simulink model "model"  (R2020a)
settings: Solver=FixedStepAuto  StartTime=0.0  StopTime=200  FixedStep=0.01  RelTol=1e-3
values from neighbouring files (symbols this model uses):
  A = zeros(5,5)    [init_test.m]
  b = 2*10^5    (= 200000)    [init_test.m]
  d1 = 2    [init_test.m]
  d2 = 3    [init_test.m]
  d3 = 3    [init_test.m]
  d4 = 2    [init_test.m]
  fleet_vel = 20    [init_test.m]
  h10 = -0.8    [init_test.m]
  h20 = h10*2    (= -1.6)    [init_test.m]
  h30 = h10*3    (= -2.4)    [init_test.m]
  h40 = h10*4    (= -3.2)    [init_test.m]
  k1 = 1.7*10^5    (= 170000)    [init_test.m]
  k2 = 1.8*10^5    (= 180000)    [init_test.m]
  k3 = 1.8*10^5    (= 180000)    [init_test.m]
  k4 = 1.2*10^5    (= 120000)    [init_test.m]
  M = 1200    [init_test.m]
  n0_init = [0 20]    [init_test.m]
  n1_init = [-10 0]    [init_test.m]
  n2_init = [-20 0]    [init_test.m]
  n3_init = [-30 0]    [init_test.m]
  n4_init = [-40 0]    [init_test.m]
  noise = 1    [init_test.m]
  u0 = 0    [init_test.m]
settings Model: Creator=mic-ciciolla  LastModifiedBy=mic-ciciolla

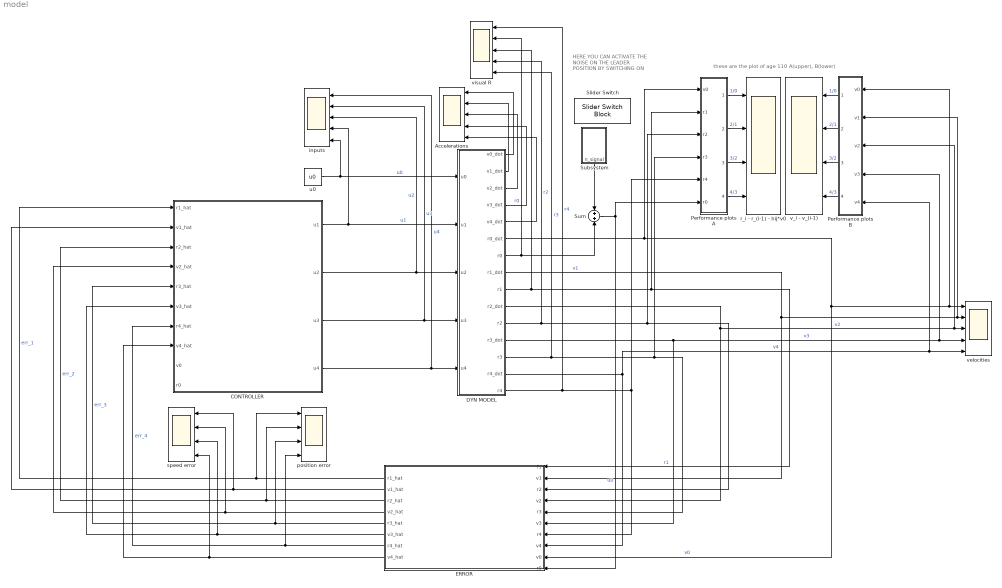
== system model ==
  note: these are the plot of age 110 A(upper), B(lower)
  note: HERE YOU CAN ACTIVATE THE NOISE ON THE LEADER POSITION BY SWITCHING ON
  Accelerations : Scope  NumInputPorts=5
  CONTROLLER : Subsystem
  DYN MODEL : Subsystem
  ERROR : Subsystem
  Performance plots A : Subsystem
  Performance plots B : Subsystem
  Slider Switch : SliderSwitchBlock
      settings: Values={{'Off', 'On'}, [0 1]}
  Subsystem : Subsystem
      settings: PortSchema="{\"entries\":[{\"content\":{\"sides\":[{\"content\":{\"connectorIds\":[]},\"type\":\"ConnectorPlacement.EquallySpacedRectSide\",\"uuid\":\"16fede81-657e-45c1-a9ae-d81e864610a5\"},{\"content\":{\"connectorIds\":[],\"side\":\"RIGHT\"},\"type\":\"ConnectorPlacement.EquallySpacedRectSide\",\"uuid\":\"97676902-59d3-4a36-b26f-8c9a1bb8a23e\"},{\"content\":{\"connectorIds\":[],\"side\":\"TOP\"},\"type\":\"ConnectorPlacement.EquallySpacedRectSide\",\"uuid\":\"8e239925-b658-4eae-ba83-be624b434eda\"},{\"content\":{\"connectorIds\":[\"Out1\"],\"side\":\"BOTTOM\"},\"type\":\"ConnectorPlacement.EquallySpacedRectSide\",\"uuid\":\"030014d3-1c2a-45c6-8ce4-97b9acd07308\"}]},\"type\":\"ConnectorPlacement.EquallySpacedConnector\",\"uuid\":\"2f76814e-6954-4e9d-8491-731c603c8c68\"}],\"packageUris\":[\"http://schema.mathworks.com/mf0/Connector/19700101\"],\"version\":\"1.0\"}"
  Sum : Sum
  inputs : Scope  NumInputPorts=5
  position error : Scope  NumInputPorts=4
  r_i - r_(i-1) - hij*v0 : Scope  NumInputPorts=4
  speed error : Scope  NumInputPorts=4
  u0 : Constant  Value=u0
  v_i - v_(i-1) : Scope  NumInputPorts=4
  velocities : Scope  NumInputPorts=5
  visual R : Scope  NumInputPorts=5
  wires:
  DYN MODEL/9(r1) -> visual R/3, Performance plots A/2(r1), ERROR/1(r1)  "r1"
  DYN MODEL/8(r1_dot) -> Performance plots B/2(v1), velocities/2, ERROR/2(v1)  "v1"
  DYN MODEL/7(r0) -> Sum/2, visual R/2  "r0"
  DYN MODEL/6(r0_dot) -> Performance plots A/1(v0), ERROR/9(v0), Performance plots B/1(v0), velocities/1  "v0"
  DYN MODEL/11(r2) -> ERROR/3(r2), Performance plots A/3(r2), visual R/4  "r2"
  DYN MODEL/10(r2_dot) -> Performance plots B/3(v2), velocities/3, ERROR/4(v2)  "v2"
  DYN MODEL/13(r3) -> ERROR/5(r3), Performance plots A/4(r3), visual R/5  "r3"
  DYN MODEL/12(r3_dot) -> Performance plots B/4(v3), velocities/4, ERROR/6(v3)  "v3"
  DYN MODEL/15(r4) -> visual R/1, Performance plots A/5(r4), ERROR/7(r4)  "r4"
  DYN MODEL/14(r4_dot) -> velocities/5, Performance plots B/5(v4), ERROR/8(v4)  "v4"
  ERROR/1(r1_hat) -> position error/1, CONTROLLER/1(r1_hat)  "err_1"
  ERROR/2(v1_hat) -> CONTROLLER/2(v1_hat), speed error/1
  ERROR/3(r2_hat) -> position error/2, CONTROLLER/3(r2_hat)  "err_2"
  ERROR/4(v2_hat) -> CONTROLLER/4(v2_hat), speed error/2
  ERROR/5(r3_hat) -> position error/3, CONTROLLER/5(r3_hat)  "err_3"
  ERROR/6(v3_hat) -> speed error/3, CONTROLLER/6(v3_hat)
  ERROR/7(r4_hat) -> position error/4, CONTROLLER/7(r4_hat)  "err_4"
  ERROR/8(v4_hat) -> speed error/4, CONTROLLER/8(v4_hat)
  CONTROLLER/1(u1) -> inputs/4, DYN MODEL/2(u1)  "u1"
  CONTROLLER/2(u2) -> inputs/3, DYN MODEL/3(u2)  "u2"
  CONTROLLER/3(u3) -> inputs/2, DYN MODEL/4(u3)  "u3"
  CONTROLLER/4(u4) -> inputs/1, DYN MODEL/5(u4)  "u4"
  Performance plots B/1(veic 1/0) -> v_i - v_(i-1)/1  "1/0"
  Performance plots B/2(veic 2/1) -> v_i - v_(i-1)/2  "2/1"
  Performance plots B/4(veic 4/3) -> v_i - v_(i-1)/4  "4/3"
  Performance plots B/3(veic 3/2) -> v_i - v_(i-1)/3  "3/2"
  Performance plots A/4(veic 4/3) -> r_i - r_(i-1) - hij*v0/4  "4/3"
  Performance plots A/3(veic 3/2) -> r_i - r_(i-1) - hij*v0/3  "3/2"
  Performance plots A/1(veic 1/0) -> r_i - r_(i-1) - hij*v0/1  "1/0"
  Performance plots A/2(veic 2/1) -> r_i - r_(i-1) - hij*v0/2  "2/1"
  u0/1 -> inputs/5, DYN MODEL/1(u0)  "u0"
  Sum/1 -> ERROR/10(r0), Performance plots A/6(r0)  "u0"
  DYN MODEL/1(v0_dot) -> Accelerations/1
  DYN MODEL/2(v1_dot) -> Accelerations/2
  DYN MODEL/3(v2_dot) -> Accelerations/3
  DYN MODEL/4(v3_dot) -> Accelerations/4
  DYN MODEL/5(v4_dot) -> Accelerations/5
  Subsystem/1(n_signal) -> Sum/1

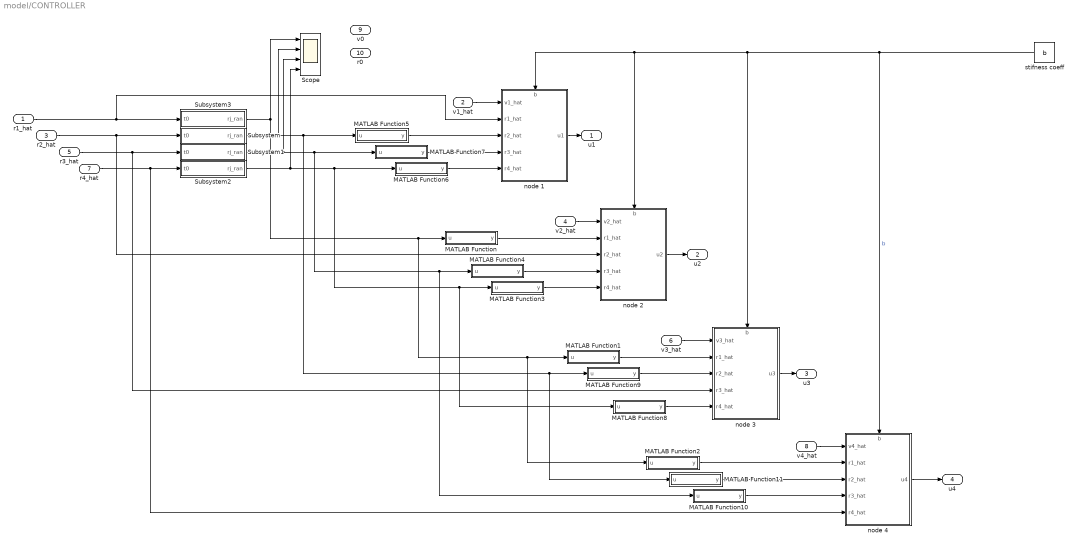
== system model/CONTROLLER ==
  r1_hat : Inport
  v1_hat : Inport  Port=2
  r2_hat : Inport  Port=3
  v2_hat : Inport  Port=4
  r3_hat : Inport  Port=5
  v3_hat : Inport  Port=6
  r4_hat : Inport  Port=7
  v4_hat : Inport  Port=8
  v0 : Inport  Port=9
  r0 : Inport  Port=10
  MATLAB Function : MATLAB Function  TreatAsAtomicUnit=on
  MATLAB Function1 : MATLAB Function  TreatAsAtomicUnit=on
  MATLAB Function10 : MATLAB Function  TreatAsAtomicUnit=on
  MATLAB Function11 : MATLAB Function  TreatAsAtomicUnit=on
  MATLAB Function2 : MATLAB Function  TreatAsAtomicUnit=on
  MATLAB Function3 : MATLAB Function  TreatAsAtomicUnit=on
  MATLAB Function4 : MATLAB Function  TreatAsAtomicUnit=on
  MATLAB Function5 : MATLAB Function  TreatAsAtomicUnit=on
  MATLAB Function6 : MATLAB Function  TreatAsAtomicUnit=on
  MATLAB Function7 : MATLAB Function  TreatAsAtomicUnit=on
  MATLAB Function8 : MATLAB Function  TreatAsAtomicUnit=on
  MATLAB Function9 : MATLAB Function  TreatAsAtomicUnit=on
  Scope : Scope  NumInputPorts=4
  Subsystem : Subsystem
  Subsystem1 : Subsystem
  Subsystem2 : Subsystem
  Subsystem3 : Subsystem
  node 1 : Subsystem
      settings: PortSchema="{\"entries\":[{\"content\":{\"sides\":[{\"content\":{\"connectorIds\":[\"In1\",\"In2\",\"In3\",\"In4\",\"In5\"]},\"type\":\"ConnectorPlacement.EquallySpacedRectSide\",\"uuid\":\"5e8ab726-83fb-4f3c-9500-0538f81a3a18\"},{\"content\":{\"connectorIds\":[\"Out1\"],\"side\":\"RIGHT\"},\"type\":\"ConnectorPlacement.EquallySpacedRectSide\",\"uuid\":\"1c3f6fdc-5897-44be-b75d-625b3a56e21f\"},{\"content\":{\"connectorIds\":[\"In6\"],\"side\":\"TOP\"},\"type\":\"ConnectorPlacement.EquallySpacedRectSide\",\"uuid\":\"dec3deb1-028d-4c92-801a-3054ae4cd420\"}]},\"type\":\"ConnectorPlacement.EquallySpacedConnector\",\"uuid\":\"f32b6f2a-1ac7-4706-92ec-1bae63a0d6a6\"}],\"packageUris\":[\"http://schema.mathworks.com/mf0/Connector/19700101\"],\"version\":\"1.0\"}"
  node 2 : Subsystem
      settings: PortSchema="{\"entries\":[{\"content\":{\"sides\":[{\"content\":{\"connectorIds\":[\"In1\",\"In2\",\"In3\",\"In4\",\"In5\"]},\"type\":\"ConnectorPlacement.EquallySpacedRectSide\",\"uuid\":\"5e8ab726-83fb-4f3c-9500-0538f81a3a18\"},{\"content\":{\"connectorIds\":[\"Out1\"],\"side\":\"RIGHT\"},\"type\":\"ConnectorPlacement.EquallySpacedRectSide\",\"uuid\":\"1c3f6fdc-5897-44be-b75d-625b3a56e21f\"},{\"content\":{\"connectorIds\":[\"In6\"],\"side\":\"TOP\"},\"type\":\"ConnectorPlacement.EquallySpacedRectSide\",\"uuid\":\"dec3deb1-028d-4c92-801a-3054ae4cd420\"}]},\"type\":\"ConnectorPlacement.EquallySpacedConnector\",\"uuid\":\"f32b6f2a-1ac7-4706-92ec-1bae63a0d6a6\"}],\"packageUris\":[\"http://schema.mathworks.com/mf0/Connector/19700101\"],\"version\":\"1.0\"}"
  node 3 : Subsystem
      settings: PortSchema="{\"entries\":[{\"content\":{\"sides\":[{\"content\":{\"connectorIds\":[\"In1\",\"In2\",\"In3\",\"In4\",\"In5\"]},\"type\":\"ConnectorPlacement.EquallySpacedRectSide\",\"uuid\":\"5e8ab726-83fb-4f3c-9500-0538f81a3a18\"},{\"content\":{\"connectorIds\":[\"Out1\"],\"side\":\"RIGHT\"},\"type\":\"ConnectorPlacement.EquallySpacedRectSide\",\"uuid\":\"1c3f6fdc-5897-44be-b75d-625b3a56e21f\"},{\"content\":{\"connectorIds\":[\"In6\"],\"side\":\"TOP\"},\"type\":\"ConnectorPlacement.EquallySpacedRectSide\",\"uuid\":\"dec3deb1-028d-4c92-801a-3054ae4cd420\"}]},\"type\":\"ConnectorPlacement.EquallySpacedConnector\",\"uuid\":\"f32b6f2a-1ac7-4706-92ec-1bae63a0d6a6\"}],\"packageUris\":[\"http://schema.mathworks.com/mf0/Connector/19700101\"],\"version\":\"1.0\"}"
  node 4 : Subsystem
      settings: PortSchema="{\"entries\":[{\"content\":{\"sides\":[{\"content\":{\"connectorIds\":[\"In1\",\"In2\",\"In3\",\"In4\",\"In5\"]},\"type\":\"ConnectorPlacement.EquallySpacedRectSide\",\"uuid\":\"5e8ab726-83fb-4f3c-9500-0538f81a3a18\"},{\"content\":{\"connectorIds\":[\"Out1\"],\"side\":\"RIGHT\"},\"type\":\"ConnectorPlacement.EquallySpacedRectSide\",\"uuid\":\"1c3f6fdc-5897-44be-b75d-625b3a56e21f\"},{\"content\":{\"connectorIds\":[\"In6\"],\"side\":\"TOP\"},\"type\":\"ConnectorPlacement.EquallySpacedRectSide\",\"uuid\":\"dec3deb1-028d-4c92-801a-3054ae4cd420\"}]},\"type\":\"ConnectorPlacement.EquallySpacedConnector\",\"uuid\":\"f32b6f2a-1ac7-4706-92ec-1bae63a0d6a6\"}],\"packageUris\":[\"http://schema.mathworks.com/mf0/Connector/19700101\"],\"version\":\"1.0\"}"
  stifness coeff : Constant  Value=b
  u1 : Outport
  u2 : Outport  Port=2
  u3 : Outport  Port=3
  u4 : Outport  Port=4
  wires:
  stifness coeff/1 -> node 1/6(b), node 2/6(b), node 3/6(b), node 4/6(b)  "b"
  v1_hat/1 -> node 1/1(v1_hat)
  node 1/1(u1) -> u1/1
  node 4/1(u4) -> u4/1
  node 3/1(u3) -> u3/1
  node 2/1(u2) -> u2/1
  v2_hat/1 -> node 2/1(v2_hat)
  v3_hat/1 -> node 3/1(v3_hat)
  v4_hat/1 -> node 4/1(v4_hat)
  r1_hat/1 -> Subsystem3/1(t0), node 1/2(r1_hat)
  r3_hat/1 -> Subsystem1/1(t0), node 3/4(r3_hat)
  r2_hat/1 -> Subsystem/1(t0), node 2/3(r2_hat)
  r4_hat/1 -> Subsystem2/1(t0), node 4/5(r4_hat)
  Subsystem/1(rj_ran) -> MATLAB Function5/1(u), MATLAB Function9/1(u), MATLAB Function11/1(u), Scope/2
  Subsystem1/1(rj_ran) -> MATLAB Function7/1(u), MATLAB Function4/1(u), MATLAB Function10/1(u), Scope/3
  Subsystem2/1(rj_ran) -> Scope/4, MATLAB Function6/1(u), MATLAB Function3/1(u), MATLAB Function8/1(u)
  Subsystem3/1(rj_ran) -> MATLAB Function/1(u), MATLAB Function1/1(u), MATLAB Function2/1(u), Scope/1
  MATLAB Function/1(y) -> node 2/2(r1_hat)
  MATLAB Function1/1(y) -> node 3/2(r1_hat)
  MATLAB Function2/1(y) -> node 4/2(r1_hat)
  MATLAB Function4/1(y) -> node 2/4(r3_hat)
  MATLAB Function3/1(y) -> node 2/5(r4_hat)
  MATLAB Function5/1(y) -> node 1/3(r2_hat)
  MATLAB Function7/1(y) -> node 1/4(r3_hat)
  MATLAB Function6/1(y) -> node 1/5(r4_hat)
  MATLAB Function9/1(y) -> node 3/3(r2_hat)
  MATLAB Function8/1(y) -> node 3/5(r4_hat)
  MATLAB Function11/1(y) -> node 4/3(r2_hat)
  MATLAB Function10/1(y) -> node 4/4(r3_hat)

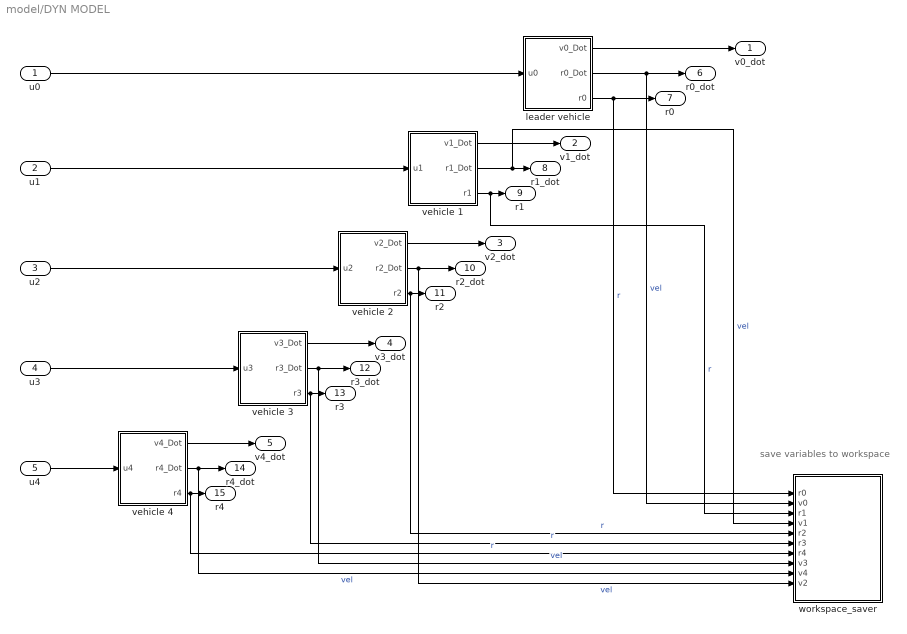
== system model/DYN MODEL ==
  note: save variables to workspace
  u0 : Inport
  u1 : Inport  Port=2
  u2 : Inport  Port=3
  u3 : Inport  Port=4
  u4 : Inport  Port=5
  leader vehicle : Subsystem
  vehicle 1 : Subsystem
  vehicle 2 : Subsystem
  vehicle 3 : Subsystem
  vehicle 4 : Subsystem
  workspace_saver : Subsystem
  v0_dot : Outport
  v1_dot : Outport  Port=2
  v2_dot : Outport  Port=3
  v3_dot : Outport  Port=4
  v4_dot : Outport  Port=5
  r0_dot : Outport  Port=6
  r0 : Outport  Port=7
  r1_dot : Outport  Port=8
  r1 : Outport  Port=9
  r2_dot : Outport  Port=10
  r2 : Outport  Port=11
  r3_dot : Outport  Port=12
  r3 : Outport  Port=13
  r4_dot : Outport  Port=14
  r4 : Outport  Port=15
  wires:
  u0/1 -> leader vehicle/1(u0)
  vehicle 4/1(v4_Dot) -> v4_dot/1
  u2/1 -> vehicle 2/1(u2)
  u4/1 -> vehicle 4/1(u4)
  u1/1 -> vehicle 1/1(u1)
  leader vehicle/1(v0_Dot) -> v0_dot/1
  vehicle 4/2(r4_Dot) -> r4_dot/1, workspace_saver/9(v4)  "vel"
  vehicle 1/1(v1_Dot) -> v1_dot/1
  vehicle 1/3(r1) -> workspace_saver/3(r1), r1/1  "r"
  leader vehicle/2(r0_Dot) -> workspace_saver/2(v0), r0_dot/1  "vel"
  vehicle 2/2(r2_Dot) -> r2_dot/1, workspace_saver/10(v2)  "vel"
  vehicle 3/1(v3_Dot) -> v3_dot/1
  vehicle 2/1(v2_Dot) -> v2_dot/1
  u3/1 -> vehicle 3/1(u3)
  vehicle 3/3(r3) -> workspace_saver/6(r3), r3/1  "r"
  vehicle 4/3(r4) -> workspace_saver/7(r4), r4/1  "r"
  vehicle 2/3(r2) -> workspace_saver/5(r2), r2/1  "r"
  vehicle 1/2(r1_Dot) -> workspace_saver/4(v1), r1_dot/1  "vel"
  vehicle 3/2(r3_Dot) -> r3_dot/1, workspace_saver/8(v3)  "vel"
  leader vehicle/3(r0) -> r0/1, workspace_saver/1(r0)  "r"

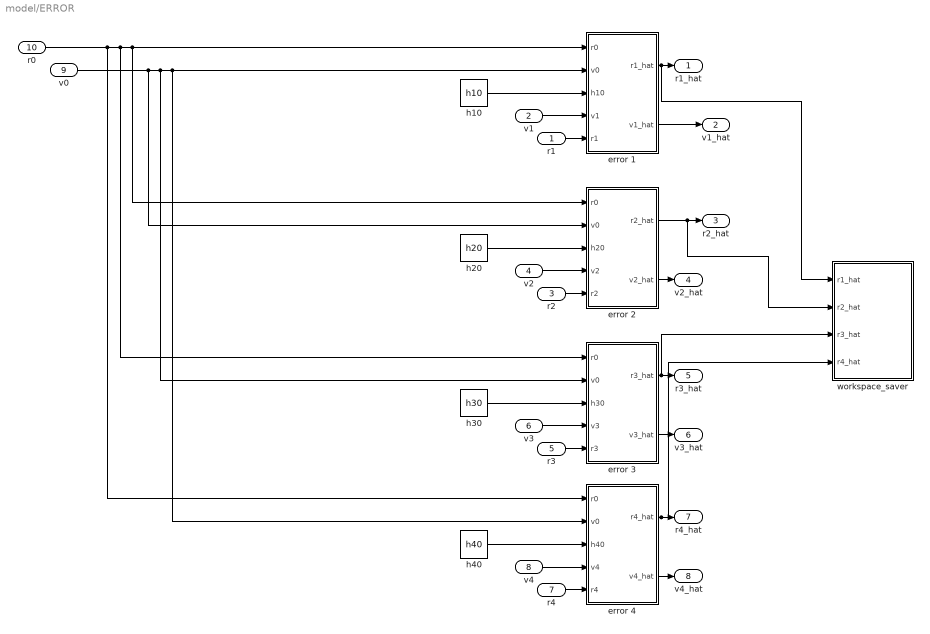
== system model/ERROR ==
  r1 : Inport
  v1 : Inport  Port=2
  r2 : Inport  Port=3
  v2 : Inport  Port=4
  r3 : Inport  Port=5
  v3 : Inport  Port=6
  r4 : Inport  Port=7
  v4 : Inport  Port=8
  v0 : Inport  Port=9
  r0 : Inport  Port=10
  error 1 : Subsystem
  error 2 : Subsystem
  error 3 : Subsystem
  error 4 : Subsystem
  h10 : Constant  Value=h10
  h20 : Constant  Value=h20
  h30 : Constant  Value=h30
  h40 : Constant  Value=h40
  workspace_saver : Subsystem
  r1_hat : Outport
  v1_hat : Outport  Port=2
  r2_hat : Outport  Port=3
  v2_hat : Outport  Port=4
  r3_hat : Outport  Port=5
  v3_hat : Outport  Port=6
  r4_hat : Outport  Port=7
  v4_hat : Outport  Port=8
  wires:
  r1/1 -> error 1/5(r1)
  r0/1 -> error 4/1(r0), error 3/1(r0), error 2/1(r0), error 1/1(r0)
  h10/1 -> error 1/3(h10)
  v1/1 -> error 1/4(v1)
  v0/1 -> error 2/2(v0), error 3/2(v0), error 4/2(v0), error 1/2(v0)
  error 1/1(r1_hat) -> workspace_saver/1(r1_hat), r1_hat/1
  error 1/2(v1_hat) -> v1_hat/1
  h20/1 -> error 2/3(h20)
  r2/1 -> error 2/5(r2)
  error 2/1(r2_hat) -> workspace_saver/2(r2_hat), r2_hat/1
  v2/1 -> error 2/4(v2)
  error 2/2(v2_hat) -> v2_hat/1
  h30/1 -> error 3/3(h30)
  r3/1 -> error 3/5(r3)
  error 3/1(r3_hat) -> workspace_saver/3(r3_hat), r3_hat/1
  v3/1 -> error 3/4(v3)
  error 3/2(v3_hat) -> v3_hat/1
  h40/1 -> error 4/3(h40)
  r4/1 -> error 4/5(r4)
  error 4/1(r4_hat) -> workspace_saver/4(r4_hat), r4_hat/1
  v4/1 -> error 4/4(v4)
  error 4/2(v4_hat) -> v4_hat/1

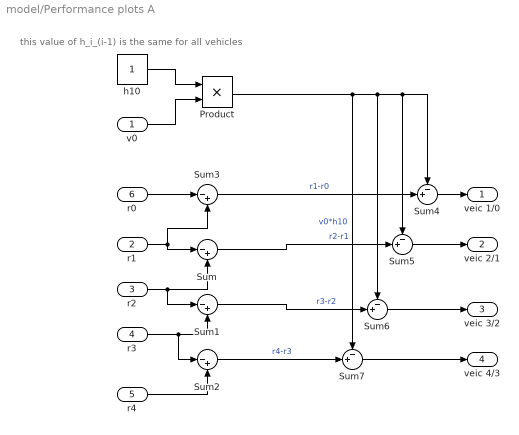
== system model/Performance plots A ==
  note: this value of h_i_(i-1) is the same for all vehicles
  v0 : Inport
  r1 : Inport  Port=2
  r2 : Inport  Port=3
  r3 : Inport  Port=4
  r4 : Inport  Port=5
  r0 : Inport  Port=6
  Product : Product
  Sum{,1..3} (4 alike) : Sum  Inputs=|-+
  Sum{4..7} (4 alike) : Sum  Inputs=-+|
  h10 : Constant
  veic 1/0 : Outport
  veic 2/1 : Outport  Port=2
  veic 3/2 : Outport  Port=3
  veic 4/3 : Outport  Port=4
  wires:
  r1/1 -> Sum3/2, Sum/1
  r2/1 -> Sum/2, Sum1/1
  h10/1 -> Product/1
  v0/1 -> Product/2
  Product/1 -> Sum4/1, Sum5/1, Sum6/1, Sum7/1  "v0*h10"
  r3/1 -> Sum2/1, Sum1/2
  r4/1 -> Sum2/2
  Sum/1 -> Sum5/2  "r2-r1"
  Sum1/1 -> Sum6/2  "r3-r2"
  Sum2/1 -> Sum7/2  "r4-r3"
  Sum3/1 -> Sum4/2  "r1-r0"
  r0/1 -> Sum3/1
  Sum4/1 -> veic 1/0/1
  Sum5/1 -> veic 2/1/1
  Sum6/1 -> veic 3/2/1
  Sum7/1 -> veic 4/3/1

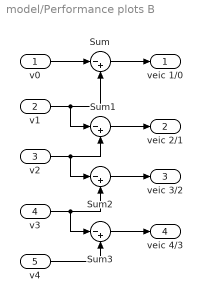
== system model/Performance plots B ==
  v0 : Inport
  v1 : Inport  Port=2
  v2 : Inport  Port=3
  v3 : Inport  Port=4
  v4 : Inport  Port=5
  Sum{,1..3} (4 alike) : Sum  Inputs=|-+
  veic 1/0 : Outport
  veic 2/1 : Outport  Port=2
  veic 3/2 : Outport  Port=3
  veic 4/3 : Outport  Port=4
  wires:
  v1/1 -> Sum/2, Sum1/1
  v0/1 -> Sum/1
  v2/1 -> Sum1/2, Sum2/1
  v3/1 -> Sum2/2, Sum3/1
  Sum/1 -> veic 1/0/1
  Sum3/1 -> veic 4/3/1
  Sum1/1 -> veic 2/1/1
  v4/1 -> Sum3/2
  Sum2/1 -> veic 3/2/1

== system model/Subsystem ==
  Clock : Clock
  MATLAB Function : MATLAB Function  TreatAsAtomicUnit=on
  noise : Constant  Value=noise
  n_signal : Outport
  wires:
  noise/1 -> MATLAB Function/2("n_signal ")
  Clock/1 -> MATLAB Function/1(time)
  MATLAB Function/1(n_signal) -> n_signal/1

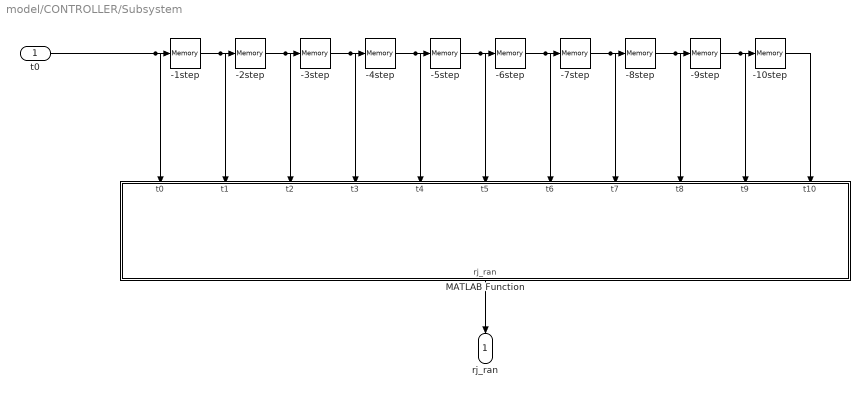
== system model/CONTROLLER/Subsystem ==
  t0 : Inport
  -10step : Memory  InitialCondition=n2_init(1)-n0_init(1)-(h20*n0_init(2))
  -1step : Memory  InitialCondition=n2_init(1)-n0_init(1)-(h20*n0_init(2))
  -2step : Memory  InitialCondition=n2_init(1)-n0_init(1)-(h20*n0_init(2))
  -3step : Memory  InitialCondition=n2_init(1)-n0_init(1)-(h20*n0_init(2))
  -4step : Memory  InitialCondition=n2_init(1)-n0_init(1)-(h20*n0_init(2))
  -5step : Memory  InitialCondition=n2_init(1)-n0_init(1)-(h20*n0_init(2))
  -6step : Memory  InitialCondition=n2_init(1)-n0_init(1)-(h20*n0_init(2))
  -7step : Memory  InitialCondition=n2_init(1)-n0_init(1)-(h20*n0_init(2))
  -8step : Memory  InitialCondition=n2_init(1)-n0_init(1)-(h20*n0_init(2))
  -9step : Memory  InitialCondition=n2_init(1)-n0_init(1)-(h20*n0_init(2))
  MATLAB Function : MATLAB Function  TreatAsAtomicUnit=on
  rj_ran : Outport
  wires:
  t0/1 -> -1step/1, MATLAB Function/1(t0)
  -1step/1 -> -2step/1, MATLAB Function/2(t1)
  -2step/1 -> MATLAB Function/3(t2), -3step/1
  -3step/1 -> -4step/1, MATLAB Function/4(t3)
  -4step/1 -> -5step/1, MATLAB Function/5(t4)
  -6step/1 -> -7step/1, MATLAB Function/7(t6)
  -7step/1 -> -8step/1, MATLAB Function/8(t7)
  -8step/1 -> -9step/1, MATLAB Function/9(t8)
  -5step/1 -> -6step/1, MATLAB Function/6(t5)
  -10step/1 -> MATLAB Function/11(t10)
  -9step/1 -> -10step/1, MATLAB Function/10(t9)
  MATLAB Function/1(rj_ran) -> rj_ran/1

== system model/CONTROLLER/Subsystem1 ==
  t0 : Inport
  -10step : Memory  InitialCondition=n3_init(1)-n0_init(1)-(h30*n0_init(2))
  -1step : Memory  InitialCondition=n3_init(1)-n0_init(1)-(h30*n0_init(2))
  -2step : Memory  InitialCondition=n3_init(1)-n0_init(1)-(h30*n0_init(2))
  -3step : Memory  InitialCondition=n3_init(1)-n0_init(1)-(h30*n0_init(2))
  -4step : Memory  InitialCondition=n3_init(1)-n0_init(1)-(h30*n0_init(2))
  -5step : Memory  InitialCondition=n3_init(1)-n0_init(1)-(h30*n0_init(2))
  -6step : Memory  InitialCondition=n3_init(1)-n0_init(1)-(h30*n0_init(2))
  -7step : Memory  InitialCondition=n3_init(1)-n0_init(1)-(h30*n0_init(2))
  -8step : Memory  InitialCondition=n3_init(1)-n0_init(1)-(h30*n0_init(2))
  -9step : Memory  InitialCondition=n3_init(1)-n0_init(1)-(h30*n0_init(2))
  MATLAB Function : MATLAB Function  TreatAsAtomicUnit=on
  rj_ran : Outport
  wires:
  t0/1 -> -1step/1, MATLAB Function/1(t0)
  -1step/1 -> -2step/1, MATLAB Function/2(t1)
  -2step/1 -> -3step/1, MATLAB Function/3(t2)
  -3step/1 -> -4step/1, MATLAB Function/4(t3)
  -4step/1 -> -5step/1, MATLAB Function/5(t4)
  -6step/1 -> -7step/1, MATLAB Function/7(t6)
  -7step/1 -> -8step/1, MATLAB Function/8(t7)
  -8step/1 -> -9step/1, MATLAB Function/9(t8)
  -5step/1 -> -6step/1, MATLAB Function/6(t5)
  -10step/1 -> MATLAB Function/11(t10)
  -9step/1 -> -10step/1, MATLAB Function/10(t9)
  MATLAB Function/1(rj_ran) -> rj_ran/1

== system model/CONTROLLER/Subsystem2 ==
  t0 : Inport
  -10step : Memory  InitialCondition=n4_init(1)-n0_init(1)-(h40*n0_init(2))
  -1step : Memory  InitialCondition=n4_init(1)-n0_init(1)-(h40*n0_init(2))
  -2step : Memory  InitialCondition=n4_init(1)-n0_init(1)-(h40*n0_init(2))
  -3step : Memory  InitialCondition=n4_init(1)-n0_init(1)-(h40*n0_init(2))
  -4step : Memory  InitialCondition=n4_init(1)-n0_init(1)-(h40*n0_init(2))
  -5step : Memory  InitialCondition=n4_init(1)-n0_init(1)-(h40*n0_init(2))
  -6step : Memory  InitialCondition=n4_init(1)-n0_init(1)-(h40*n0_init(2))
  -7step : Memory  InitialCondition=n4_init(1)-n0_init(1)-(h40*n0_init(2))
  -8step : Memory  InitialCondition=n4_init(1)-n0_init(1)-(h40*n0_init(2))
  -9step : Memory  InitialCondition=n4_init(1)-n0_init(1)-(h40*n0_init(2))
  MATLAB Function : MATLAB Function  TreatAsAtomicUnit=on
  rj_ran : Outport
  wires:
  t0/1 -> -1step/1, MATLAB Function/1(t0)
  -1step/1 -> -2step/1, MATLAB Function/2(t1)
  -2step/1 -> -3step/1, MATLAB Function/3(t2)
  -3step/1 -> -4step/1, MATLAB Function/4(t3)
  -4step/1 -> -5step/1, MATLAB Function/5(t4)
  -6step/1 -> -7step/1, MATLAB Function/7(t6)
  -7step/1 -> -8step/1, MATLAB Function/8(t7)
  -8step/1 -> -9step/1, MATLAB Function/9(t8)
  -5step/1 -> -6step/1, MATLAB Function/6(t5)
  -10step/1 -> MATLAB Function/11(t10)
  -9step/1 -> -10step/1, MATLAB Function/10(t9)
  MATLAB Function/1(rj_ran) -> rj_ran/1

== system model/CONTROLLER/Subsystem3 ==
  t0 : Inport
  -10step : Memory  InitialCondition=n1_init(1)-n0_init(1)-(h10*n0_init(2))
  -1step : Memory  InitialCondition=n1_init(1)-n0_init(1)-(h10*n0_init(2))
  -2step : Memory  InitialCondition=n1_init(1)-n0_init(1)-(h10*n0_init(2))
  -3step : Memory  InitialCondition=n1_init(1)-n0_init(1)-(h10*n0_init(2))
  -4step : Memory  InitialCondition=n1_init(1)-n0_init(1)-(h10*n0_init(2))
  -5step : Memory  InitialCondition=n1_init(1)-n0_init(1)-(h10*n0_init(2))
  -6step : Memory  InitialCondition=n1_init(1)-n0_init(1)-(h10*n0_init(2))
  -7step : Memory  InitialCondition=n1_init(1)-n0_init(1)-(h10*n0_init(2))
  -8step : Memory  InitialCondition=n1_init(1)-n0_init(1)-(h10*n0_init(2))
  -9step : Memory  InitialCondition=n1_init(1)-n0_init(1)-(h10*n0_init(2))
  MATLAB Function : MATLAB Function  TreatAsAtomicUnit=on
  rj_ran : Outport
  wires:
  t0/1 -> -1step/1, MATLAB Function/1(t0)
  -1step/1 -> -2step/1, MATLAB Function/2(t1)
  -2step/1 -> MATLAB Function/3(t2), -3step/1
  -3step/1 -> -4step/1, MATLAB Function/4(t3)
  -4step/1 -> -5step/1, MATLAB Function/5(t4)
  -6step/1 -> -7step/1, MATLAB Function/7(t6)
  -7step/1 -> -8step/1, MATLAB Function/8(t7)
  -8step/1 -> -9step/1, MATLAB Function/9(t8)
  -5step/1 -> -6step/1, MATLAB Function/6(t5)
  -10step/1 -> MATLAB Function/11(t10)
  -9step/1 -> -10step/1, MATLAB Function/10(t9)
  MATLAB Function/1(rj_ran) -> rj_ran/1

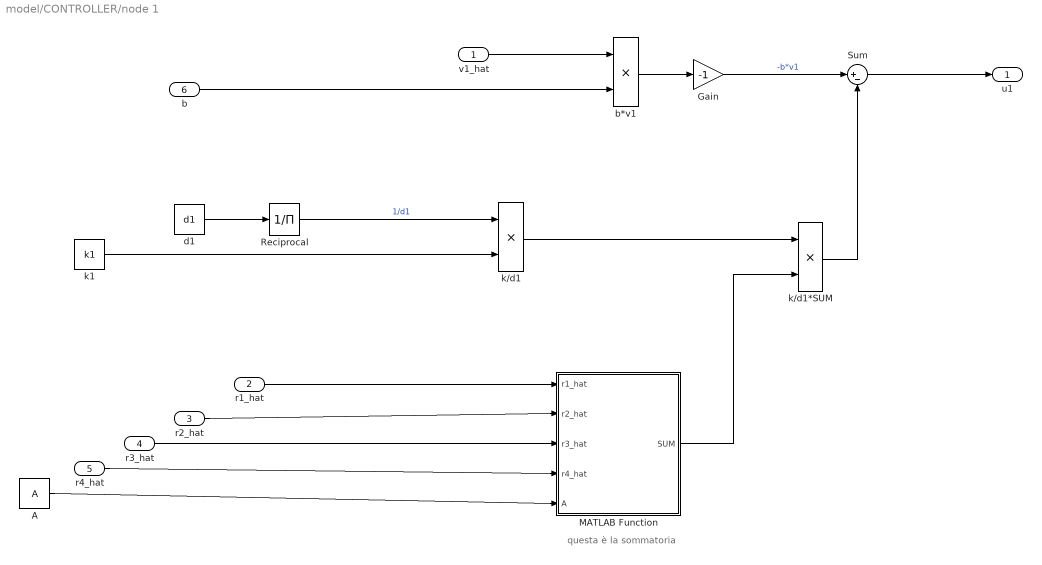
== system model/CONTROLLER/node 1 ==
  note: questa è la sommatoria
  v1_hat : Inport
  r1_hat : Inport  Port=2
  r2_hat : Inport  Port=3
  r3_hat : Inport  Port=4
  r4_hat : Inport  Port=5
  b : Inport  Port=6
  A : Constant  Value=A
  Gain : Gain  Gain=-1
  MATLAB Function : MATLAB Function  TreatAsAtomicUnit=on
  Reciprocal : Product  Inputs=/
  Sum : Sum  Inputs=|+-
  b*v1 : Product
  d1 : Constant  Value=d1
  k/d1 : Product
  k/d1*SUM : Product
  k1 : Constant  Value=k1
  u1 : Outport
  wires:
  b*v1/1 -> Gain/1
  b/1 -> b*v1/2
  Gain/1 -> Sum/1  "-b*v1"
  Sum/1 -> u1/1
  v1_hat/1 -> b*v1/1
  d1/1 -> Reciprocal/1
  Reciprocal/1 -> k/d1/1  "1/d1"
  k1/1 -> k/d1/2
  k/d1/1 -> k/d1*SUM/1
  k/d1*SUM/1 -> Sum/2
  r1_hat/1 -> MATLAB Function/1(r1_hat)
  r2_hat/1 -> MATLAB Function/2(r2_hat)
  r3_hat/1 -> MATLAB Function/3(r3_hat)
  r4_hat/1 -> MATLAB Function/4(r4_hat)
  A/1 -> MATLAB Function/5(A)
  MATLAB Function/1(SUM) -> k/d1*SUM/2

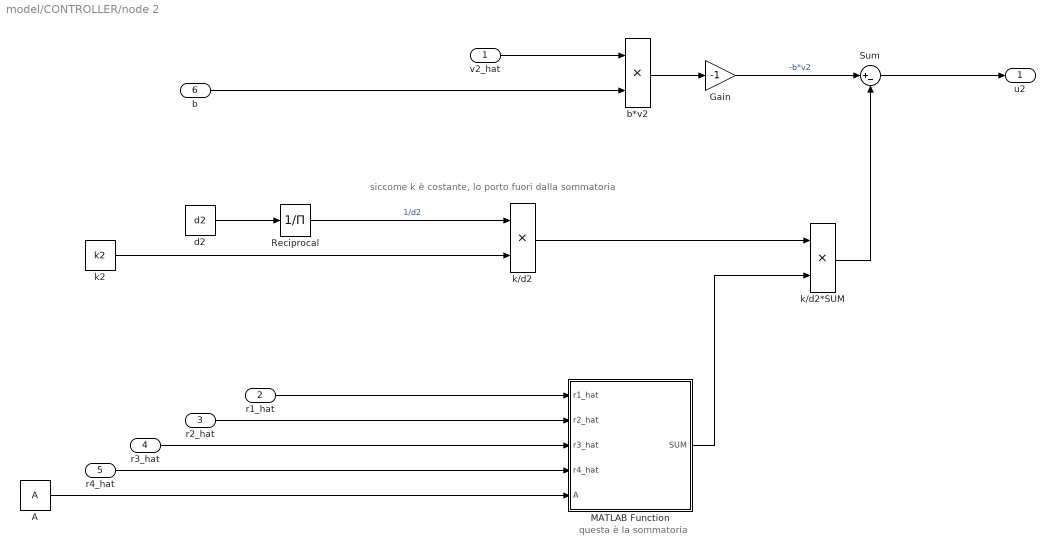
== system model/CONTROLLER/node 2 ==
  note: questa è la sommatoria
  note: siccome k è costante, lo porto fuori dalla sommatoria
  v2_hat : Inport
  r1_hat : Inport  Port=2
  r2_hat : Inport  Port=3
  r3_hat : Inport  Port=4
  r4_hat : Inport  Port=5
  b : Inport  Port=6
  A : Constant  Value=A
  Gain : Gain  Gain=-1
  MATLAB Function : MATLAB Function  TreatAsAtomicUnit=on
  Reciprocal : Product  Inputs=/
  Sum : Sum  Inputs=|+-
  b*v2 : Product
  d2 : Constant  Value=d2
  k/d2 : Product
  k/d2*SUM : Product
  k2 : Constant  Value=k2
  u2 : Outport
  wires:
  b*v2/1 -> Gain/1
  b/1 -> b*v2/2
  Gain/1 -> Sum/1  "-b*v2"
  Sum/1 -> u2/1
  v2_hat/1 -> b*v2/1
  d2/1 -> Reciprocal/1
  Reciprocal/1 -> k/d2/1  "1/d2"
  k2/1 -> k/d2/2
  k/d2/1 -> k/d2*SUM/1
  k/d2*SUM/1 -> Sum/2
  r1_hat/1 -> MATLAB Function/1(r1_hat)
  r2_hat/1 -> MATLAB Function/2(r2_hat)
  r3_hat/1 -> MATLAB Function/3(r3_hat)
  r4_hat/1 -> MATLAB Function/4(r4_hat)
  A/1 -> MATLAB Function/5(A)
  MATLAB Function/1(SUM) -> k/d2*SUM/2

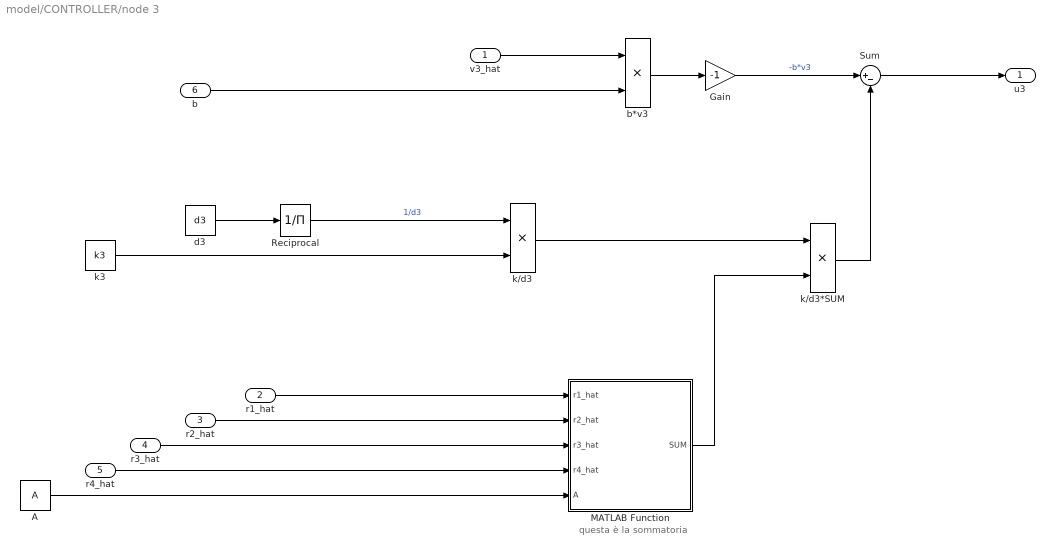
== system model/CONTROLLER/node 3 ==
  note: questa è la sommatoria
  v3_hat : Inport
  r1_hat : Inport  Port=2
  r2_hat : Inport  Port=3
  r3_hat : Inport  Port=4
  r4_hat : Inport  Port=5
  b : Inport  Port=6
  A : Constant  Value=A
  Gain : Gain  Gain=-1
  MATLAB Function : MATLAB Function  TreatAsAtomicUnit=on
  Reciprocal : Product  Inputs=/
  Sum : Sum  Inputs=|+-
  b*v3 : Product
  d3 : Constant  Value=d3
  k/d3 : Product
  k/d3*SUM : Product
  k3 : Constant  Value=k3
  u3 : Outport
  wires:
  b*v3/1 -> Gain/1
  b/1 -> b*v3/2
  Gain/1 -> Sum/1  "-b*v3"
  Sum/1 -> u3/1
  v3_hat/1 -> b*v3/1
  d3/1 -> Reciprocal/1
  Reciprocal/1 -> k/d3/1  "1/d3"
  k3/1 -> k/d3/2
  k/d3/1 -> k/d3*SUM/1
  k/d3*SUM/1 -> Sum/2
  r1_hat/1 -> MATLAB Function/1(r1_hat)
  r2_hat/1 -> MATLAB Function/2(r2_hat)
  r3_hat/1 -> MATLAB Function/3(r3_hat)
  r4_hat/1 -> MATLAB Function/4(r4_hat)
  A/1 -> MATLAB Function/5(A)
  MATLAB Function/1(SUM) -> k/d3*SUM/2

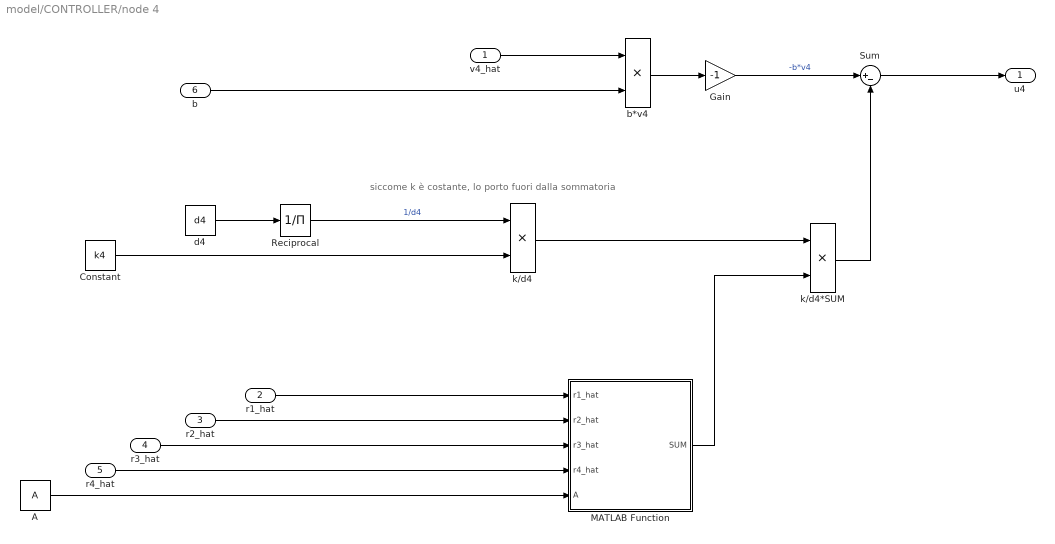
== system model/CONTROLLER/node 4 ==
  note: siccome k è costante, lo porto fuori dalla sommatoria
  v4_hat : Inport
  r1_hat : Inport  Port=2
  r2_hat : Inport  Port=3
  r3_hat : Inport  Port=4
  r4_hat : Inport  Port=5
  b : Inport  Port=6
  A : Constant  Value=A
  Constant : Constant  Value=k4  VectorParams1D=off
  Gain : Gain  Gain=-1
  MATLAB Function : MATLAB Function  TreatAsAtomicUnit=on
  Reciprocal : Product  Inputs=/
  Sum : Sum  Inputs=|+-
  b*v4 : Product
  d4 : Constant  Value=d4
  k/d4 : Product
  k/d4*SUM : Product
  u4 : Outport
  wires:
  b*v4/1 -> Gain/1
  b/1 -> b*v4/2
  Gain/1 -> Sum/1  "-b*v4"
  Sum/1 -> u4/1
  v4_hat/1 -> b*v4/1
  d4/1 -> Reciprocal/1
  Reciprocal/1 -> k/d4/1  "1/d4"
  k/d4/1 -> k/d4*SUM/1
  k/d4*SUM/1 -> Sum/2
  r1_hat/1 -> MATLAB Function/1(r1_hat)
  r2_hat/1 -> MATLAB Function/2(r2_hat)
  r3_hat/1 -> MATLAB Function/3(r3_hat)
  r4_hat/1 -> MATLAB Function/4(r4_hat)
  A/1 -> MATLAB Function/5(A)
  MATLAB Function/1(SUM) -> k/d4*SUM/2
  Constant/1 -> k/d4/2

== system model/DYN MODEL/leader vehicle ==
  u0 : Inport
  Integrator : Integrator  InitialCondition=n0_init(2)
  Integrator1 : Integrator  InitialCondition=n0_init(1)
  M : Constant  Value=M
  Product : Product
  Reciprocal : Product  Inputs=/
  Scope : Scope
  "saturation and exponential growth to \"fleet_vel\" constant" : Subsystem
  v0_Dot : Outport
  r0_Dot : Outport  Port=2
  r0 : Outport  Port=3
  wires:
  Product/1 -> Integrator/1, v0_Dot/1  "v0_Dot"
  Integrator1/1 -> r0/1
  Reciprocal/1 -> Product/1  "1/M"
  M/1 -> Reciprocal/1
  u0/1 -> Product/2
  Integrator/1 -> Integrator1/1, Scope/1, r0_Dot/1  "leader_velocity"

== system model/DYN MODEL/vehicle 1 ==
  u1 : Inport
  Integrator : Integrator  InitialCondition=n1_init(2)
  Integrator1 : Integrator  InitialCondition=n1_init(1)
  M : Constant  Value=M
  Product : Product
  Reciprocal : Product  Inputs=/
  v1_Dot : Outport
  r1_Dot : Outport  Port=2
  r1 : Outport  Port=3
  wires:
  u1/1 -> Product/2
  Reciprocal/1 -> Product/1  "1/M"
  Product/1 -> Integrator/1, v1_Dot/1  "v1_Dot"
  M/1 -> Reciprocal/1
  Integrator/1 -> Integrator1/1, r1_Dot/1  "r1_Dot"
  Integrator1/1 -> r1/1

== system model/DYN MODEL/vehicle 2 ==
  u2 : Inport
  Integrator : Integrator  InitialCondition=n2_init(2)
  Integrator1 : Integrator  InitialCondition=n2_init(1)
  M : Constant  Value=M
  Product : Product
  Reciprocal : Product  Inputs=/
  v2_Dot : Outport
  r2_Dot : Outport  Port=2
  r2 : Outport  Port=3
  wires:
  u2/1 -> Product/2
  Reciprocal/1 -> Product/1  "1/M"
  Product/1 -> Integrator/1, v2_Dot/1  "v2_Dot"
  M/1 -> Reciprocal/1
  Integrator/1 -> Integrator1/1, r2_Dot/1  "r2_Dot"
  Integrator1/1 -> r2/1

== system model/DYN MODEL/vehicle 3 ==
  u3 : Inport
  Integrator : Integrator  InitialCondition=n3_init(2)
  Integrator1 : Integrator  InitialCondition=n3_init(1)
  M : Constant  Value=M
  Product : Product
  Reciprocal : Product  Inputs=/
  v3_Dot : Outport
  r3_Dot : Outport  Port=2
  r3 : Outport  Port=3
  wires:
  u3/1 -> Product/2
  Reciprocal/1 -> Product/1  "1/M"
  Product/1 -> Integrator/1, v3_Dot/1  "v3_Dot"
  M/1 -> Reciprocal/1
  Integrator/1 -> Integrator1/1, r3_Dot/1  "r3_Dot"
  Integrator1/1 -> r3/1

== system model/DYN MODEL/vehicle 4 ==
  u4 : Inport
  Integrator : Integrator  InitialCondition=n4_init(2)
  Integrator1 : Integrator  InitialCondition=n4_init(1)
  M : Constant  Value=M
  Product : Product
  Reciprocal : Product  Inputs=/
  v4_Dot : Outport
  r4_Dot : Outport  Port=2
  r4 : Outport  Port=3
  wires:
  u4/1 -> Product/2
  Reciprocal/1 -> Product/1  "1/M"
  Product/1 -> Integrator/1, v4_Dot/1  "v4_Dot"
  M/1 -> Reciprocal/1
  Integrator/1 -> Integrator1/1, r4_Dot/1  "r4_Dot"
  Integrator1/1 -> r4/1

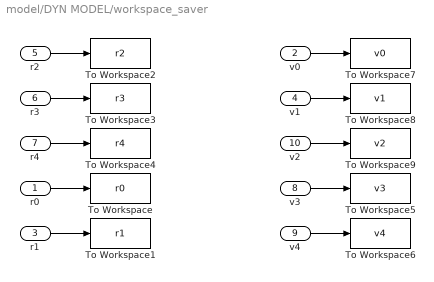
== system model/DYN MODEL/workspace_saver ==
  r0 : Inport
  v0 : Inport  Port=2
  r1 : Inport  Port=3
  v1 : Inport  Port=4
  r2 : Inport  Port=5
  r3 : Inport  Port=6
  r4 : Inport  Port=7
  v3 : Inport  Port=8
  v4 : Inport  Port=9
  v2 : Inport  Port=10
  To Workspace : ToWorkspace  VariableName=r0  SaveFormat=Structure With Time  SampleTime=-1
  To Workspace1 : ToWorkspace  VariableName=r1  SampleTime=-1
  To Workspace2 : ToWorkspace  VariableName=r2  SampleTime=-1
  To Workspace3 : ToWorkspace  VariableName=r3  SampleTime=-1
  To Workspace4 : ToWorkspace  VariableName=r4  SampleTime=-1
  To Workspace5 : ToWorkspace  VariableName=v3  SampleTime=-1
  To Workspace6 : ToWorkspace  VariableName=v4  SampleTime=-1
  To Workspace7 : ToWorkspace  VariableName=v0  SampleTime=-1
  To Workspace8 : ToWorkspace  VariableName=v1  SampleTime=-1
  To Workspace9 : ToWorkspace  VariableName=v2  SampleTime=-1
  wires:
  r4/1 -> To Workspace4/1
  r2/1 -> To Workspace2/1
  r3/1 -> To Workspace3/1
  r1/1 -> To Workspace1/1
  r0/1 -> To Workspace/1
  v2/1 -> To Workspace9/1
  v4/1 -> To Workspace6/1
  v0/1 -> To Workspace7/1
  v1/1 -> To Workspace8/1
  v3/1 -> To Workspace5/1

== system model/ERROR/error 1 ==
  r0 : Inport
  v0 : Inport  Port=2
  h10 : Inport  Port=3
  v1 : Inport  Port=4
  r1 : Inport  Port=5
  Product : Product
  Sum : Sum  Inputs=|+-
  Sum4 : Sum  Inputs=|+--
  r1_hat : Outport
  v1_hat : Outport  Port=2
  wires:
  h10/1 -> Product/1
  r1/1 -> Sum4/1
  Sum/1 -> v1_hat/1  "v1-v0"
  Product/1 -> Sum4/3
  r0/1 -> Sum4/2
  v0/1 -> Product/2, Sum/2
  v1/1 -> Sum/1
  Sum4/1 -> r1_hat/1

== system model/ERROR/error 2 ==
  r0 : Inport
  v0 : Inport  Port=2
  h20 : Inport  Port=3
  v2 : Inport  Port=4
  r2 : Inport  Port=5
  Product : Product
  Sum : Sum  Inputs=|+-
  Sum4 : Sum  Inputs=|+--
  r2_hat : Outport
  v2_hat : Outport  Port=2
  wires:
  h20/1 -> Product/1
  r2/1 -> Sum4/1
  Sum/1 -> v2_hat/1  "v2-v0"
  Product/1 -> Sum4/3
  r0/1 -> Sum4/2
  v0/1 -> Product/2, Sum/2
  v2/1 -> Sum/1
  Sum4/1 -> r2_hat/1

== system model/ERROR/error 3 ==
  r0 : Inport
  v0 : Inport  Port=2
  h30 : Inport  Port=3
  v3 : Inport  Port=4
  r3 : Inport  Port=5
  Product : Product
  Sum : Sum  Inputs=|+-
  Sum4 : Sum  Inputs=|+--
  r3_hat : Outport
  v3_hat : Outport  Port=2
  wires:
  h30/1 -> Product/1
  r3/1 -> Sum4/1
  Sum/1 -> v3_hat/1  "v3-v0"
  Product/1 -> Sum4/3
  r0/1 -> Sum4/2
  v0/1 -> Product/2, Sum/2
  v3/1 -> Sum/1
  Sum4/1 -> r3_hat/1

== system model/ERROR/error 4 ==
  r0 : Inport
  v0 : Inport  Port=2
  h40 : Inport  Port=3
  v4 : Inport  Port=4
  r4 : Inport  Port=5
  Product : Product
  Sum : Sum  Inputs=|+-
  Sum4 : Sum  Inputs=|+--
  r4_hat : Outport
  v4_hat : Outport  Port=2
  wires:
  h40/1 -> Product/1
  r4/1 -> Sum4/1
  Sum/1 -> v4_hat/1  "v4-v0"
  Product/1 -> Sum4/3
  r0/1 -> Sum4/2
  v0/1 -> Product/2, Sum/2
  v4/1 -> Sum/1
  Sum4/1 -> r4_hat/1

== system model/ERROR/workspace_saver ==
  r1_hat : Inport
  r2_hat : Inport  Port=2
  r3_hat : Inport  Port=3
  r4_hat : Inport  Port=4
  To Workspace : ToWorkspace  VariableName=err40  SampleTime=-1
  To Workspace2 : ToWorkspace  VariableName=err10  SampleTime=-1
  To Workspace3 : ToWorkspace  VariableName=err20  SampleTime=-1
  To Workspace4 : ToWorkspace  VariableName=err30  SampleTime=-1
  wires:
  r3_hat/1 -> To Workspace4/1
  r1_hat/1 -> To Workspace2/1
  r2_hat/1 -> To Workspace3/1
  r4_hat/1 -> To Workspace/1

== system model/DYN MODEL/leader vehicle/saturation and exponential growth to "fleet_vel" constant ==
  v : Inport
  Clock : Clock
  MATLAB Function : MATLAB Function  TreatAsAtomicUnit=on
  Scope1 : Scope  NumInputPorts=2
  fleet_vel : Constant  Value=fleet_vel
  v_new : Outport
  wires:
  MATLAB Function/1(v0_new) -> Scope1/2
  fleet_vel/1 -> Scope1/1, MATLAB Function/1(fleet_vel)
  v/1 -> MATLAB Function/2(v)
  Clock/1 -> MATLAB Function/3(time)

== matlab function model/CONTROLLER/Subsystem2/MATLAB Function ==
  settings: updateMethod=DISCRETE  sampleTime=0.01
  data: t0 input; rj_ran output; t1 input; t2 input; t3 input; t4 input; t5 input; t6 input; t7 input; t8 input; t9 input; t10 input
function rj_ran = fcn(t0,t1,t2,t3,t4,t5,t6,t7,t8,t9,t10)
rj_ran = [t0,t1,t2,t3,t4,t5,t6,t7,t8,t9,t10];
%rj_ran = ar(1);
%rj_ran = ar(randi([1,11]));
end

== matlab function model/CONTROLLER/Subsystem3/MATLAB Function ==
  settings: updateMethod=DISCRETE  sampleTime=0.01
  data: t0 input; rj_ran output; t1 input; t2 input; t3 input; t4 input; t5 input; t6 input; t7 input; t8 input; t9 input; t10 input
function rj_ran = fcn(t0,t1,t2,t3,t4,t5,t6,t7,t8,t9,t10)
rj_ran = [t0,t1,t2,t3,t4,t5,t6,t7,t8,t9,t10];
%i=randi([1,11]);
%rj_ran = ar(i);
%rj_ran = ar(randi([1,11]));
end

== matlab function model/CONTROLLER/MATLAB Function ==
  data: u input; y output
function y = fcn(u)

y = u(randi([1,11]));
end

== matlab function model/CONTROLLER/MATLAB Function1 ==
  data: u input; y output
function y = fcn(u)

y = u(randi([1,11]));
end

== matlab function model/CONTROLLER/MATLAB Function2 ==
  data: u input; y output
function y = fcn(u)

y = u(randi([1,11]));
end

== matlab function model/CONTROLLER/MATLAB Function3 ==
  data: u input; y output
function y = fcn(u)

y = u(randi([1,11]));
end

== matlab function model/CONTROLLER/node 2/MATLAB Function ==
  data: r1_hat input; SUM output; r2_hat input; r3_hat input; r4_hat input; A input
function SUM = getSum(r1_hat, r2_hat, r3_hat, r4_hat, A)


SUM = r2_hat*A(3,1) + A(3,2)*(r2_hat - r1_hat) + A(3,4)*(r2_hat - r3_hat) + A(3,5)*(r2_hat - r4_hat);
end

== matlab function model/CONTROLLER/MATLAB Function4 ==
  data: u input; y output
function y = fcn(u)

y = u(randi([1,11]));
end

== matlab function model/CONTROLLER/MATLAB Function5 ==
  data: u input; y output
function y = fcn(u)

y = u(randi([1,11]));
end

== matlab function model/CONTROLLER/MATLAB Function6 ==
  data: u input; y output
function y = fcn(u)

y = u(randi([1,11]));
end

== matlab function model/CONTROLLER/MATLAB Function7 ==
  data: u input; y output
function y = fcn(u)

y = u(randi([1,11]));
end

== matlab function model/CONTROLLER/MATLAB Function8 ==
  data: u input; y output
function y = fcn(u)

y = u(randi([1,11]));
end

== matlab function model/CONTROLLER/MATLAB Function9 ==
  data: u input; y output
function y = fcn(u)

y = u(randi([1,11]));
end

== matlab function model/CONTROLLER/MATLAB Function10 ==
  data: u input; y output
function y = fcn(u)

y = u(randi([1,11]));
end

== matlab function model/CONTROLLER/MATLAB Function11 ==
  data: u input; y output
function y = fcn(u)

y = u(randi([1,11]));
end

== matlab function model/CONTROLLER/node 1/MATLAB Function ==
  data: r1_hat input; SUM output; r2_hat input; r3_hat input; r4_hat input; A input
function SUM = getSum(r1_hat, r2_hat, r3_hat, r4_hat, A)

% a10 is the second row - first column element = a21
% same reason for a12, a13, a14.

% first element is a10*(r1_hat - r0_hat) but r0_hat==0
SUM = r1_hat*A(2,1) + A(2,3)*(r1_hat- r2_hat) + A(2,4)*(r1_hat - r3_hat) + A(2,5)*(r1_hat - r4_hat);

end

== matlab function model/CONTROLLER/node 3/MATLAB Function ==
  data: r1_hat input; SUM output; r2_hat input; r3_hat input; r4_hat input; A input
function SUM = getSum(r1_hat, r2_hat, r3_hat, r4_hat, A)


SUM = r3_hat*A(4,1) + A(4,2)*(r3_hat - r1_hat) + A(4,3)*(r3_hat - r2_hat) + A(4,5)*(r3_hat - r4_hat);
end

== matlab function model/CONTROLLER/node 4/MATLAB Function ==
  data: r1_hat input; SUM output; r2_hat input; r3_hat input; r4_hat input; A input
function SUM = getSum(r1_hat, r2_hat, r3_hat, r4_hat, A)


SUM = r4_hat*A(5,1) + A(5,2)*(r4_hat - r1_hat) + A(5,3)*(r4_hat - r2_hat) + A(5,4)*(r4_hat - r3_hat);
end

== matlab function model/Subsystem/MATLAB Function ==
  data: time input; n_signal output; n_signal input
function n_signal = sinusoidal_noise(time, n_signal)

if n_signal == 1 && time > 49.9

    w = pi/5;
    A = 4;

    n_signal = A*sin(w*time);
else n_signal = 0;
end

== matlab function model/DYN MODEL/leader vehicle/saturation and exponential growth to "fleet_vel" constant/MATLAB Function ==
  data: fleet_vel input; v0_new output; v input; time input
function v0_new = fcn(fleet_vel, v, time)

v0_new = fleet_vel - time*(fleet_vel - v);
end

== matlab function model/CONTROLLER/Subsystem/MATLAB Function ==
  settings: updateMethod=DISCRETE  sampleTime=0.01
  data: t0 input; rj_ran output; t1 input; t2 input; t3 input; t4 input; t5 input; t6 input; t7 input; t8 input; t9 input; t10 input
function rj_ran = fcn(t0,t1,t2,t3,t4,t5,t6,t7,t8,t9,t10)
rj_ran = [t0,t1,t2,t3,t4,t5,t6,t7,t8,t9,t10];
%i=randi([1,11]);
%rj_ran = ar(i);
%rj_ran = ar(randi([1,11]));
end

== matlab function model/CONTROLLER/Subsystem1/MATLAB Function ==
  settings: updateMethod=DISCRETE  sampleTime=0.01
  data: t0 input; rj_ran output; t1 input; t2 input; t3 input; t4 input; t5 input; t6 input; t7 input; t8 input; t9 input; t10 input
function rj_ran = fcn(t0,t1,t2,t3,t4,t5,t6,t7,t8,t9,t10)
rj_ran = [t0,t1,t2,t3,t4,t5,t6,t7,t8,t9,t10];
%rj_ran = ar(1);
%rj_ran = ar(randi([1,11]));
end
